simulink model "aufgabe_9_sim"  (R2016b)
settings: Solver=VariableStepAuto  StartTime=0.0  StopTime=10  RelTol=1e-3
libraries: cstblocks x5, simulink x1
settings Model: Creator=M  LastModifiedBy=M

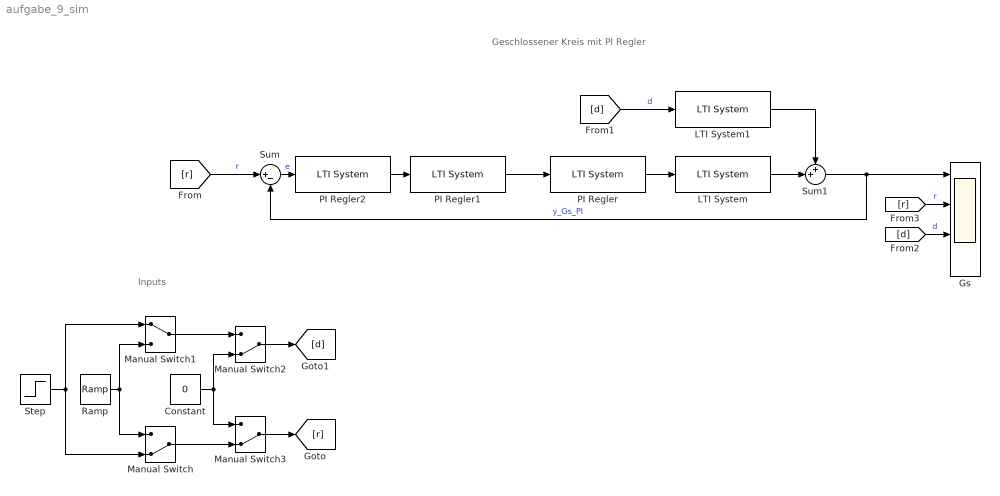
== system aufgabe_9_sim ==
  note: Inputs
  note: Geschlossener Kreis mit PI Regler
  Constant : Constant  Value=0
  Gs : Scope  NumInputPorts=4
  LTI System : cstblocks/LTI System  sys=Gs  IC=[]
  LTI System1 : cstblocks/LTI System  sys=0  IC=[]
  Manual Switch : ManualSwitch  CurrentSetting=0
  Manual Switch1 : ManualSwitch
  Manual Switch2 : ManualSwitch  CurrentSetting=0
  Manual Switch3 : ManualSwitch  CurrentSetting=0
  PI Regler : cstblocks/LTI System  sys=R_lag  IC=[]
  PI Regler1 : cstblocks/LTI System  sys=R_lead  IC=[]
  PI Regler2 : cstblocks/LTI System  sys=V_R  IC=[]
  Ramp : simulink/Sources/Ramp  slope=1  start=1  X0=0
  Step : Step  SampleTime=0
  Sum : Sum  Inputs=|+-
  Sum1 : Sum  Inputs=++|
  wires:
  PI Regler/1 -> LTI System/1
  LTI System1/1 -> Sum1/1
  LTI System/1 -> Sum1/2
  Sum1/1 -> Sum/2, Gs/1  "y_Gs_PI"
  Manual Switch1/1 -> Manual Switch2/1
  Constant/1 -> Manual Switch3/1, Manual Switch2/2
  Manual Switch2/1 -> [d]
  [d] -> LTI System1/1  "d"
  [r] -> Sum/1  "r"
  Manual Switch3/1 -> [r]
  Manual Switch/1 -> Manual Switch3/2
  Ramp/1 -> Manual Switch/1, Manual Switch1/2
  Step/1 -> Manual Switch/2, Manual Switch1/1
  [d] -> Gs/3  "d"
  [r] -> Gs/2  "r"
  PI Regler1/1 -> PI Regler/1
  PI Regler2/1 -> PI Regler1/1
  Sum/1 -> PI Regler2/1  "e"
